simulink library "speedgoatlib_IO622"  (R2024b)
settings: Solver=ode45  StartTime=0.0  StopTime=10.0  RelTol=1e-3  EnableMultiTasking=on
libraries: slrealtimeethercatlib x10, simulink x4, simulink_extras x2
Description:
  | 7.14.0.739 (R2012a)
settings Model: sg_rtwmakecfg_data=_sglibc_  Creator=dkuratli  LastModifiedBy=speedgoat\jenkins
settings SolverCC: AlgebraicLoopSolver=TrustRegion
settings DataIOCC: LimitDataPoints=on  SaveFormat=Array  SignalLoggingSaveFormat=ModelDataLogs  ReturnWorkspaceOutputs=off
settings OptimizationCC: ReuseModelBlockBuffer=off  ExpressionDepthLimit=2147483647  LifeSpan=inf
settings DebuggingCC: UnderspecifiedInitializationDetection=Classic  MergeDetectMultiDrivingBlocksExec=none  SolverPrmCheckMsg=warning  FcnCallInpInsideContextMsg=warning  UnconnectedInputMsg=warning  UnconnectedOutputMsg=warning  UnconnectedLineMsg=warning  AllowSymbolicDim=off  StateNameClashWarn=warning  PregeneratedLibrarySubsystemCodeDiagnostic=none  SFUnexpectedBacktrackingDiag=warning  SFNoUnconditionalDefaultTransitionDiag=warning  SFExecutionAtInitializationDiag=none  ArithmeticOperatorsInVariantConditions=warning
settings HardwareCC: ProdBitPerPointer=32  ProdBitPerSizeT=32  ProdBitPerPtrDiffT=32  ProdLargestAtomicFloat=None  ProdIntDivRoundTo=Undefined  ProdEndianess=Unspecified  ProdWordSize=32  ProdHWDeviceType=32-bit Generic
settings ModelReferenceCC: EnableRefExpFcnMdlSchedulingChecks=on  PropagateSignalLabelsOutOfModel=off
settings SFSimCC: SimUseLocalCustomCode=off  CustomCodeUndefinedFunction=UseInterfaceOnly
settings RTWCC: RTWUseLocalCustomCode=off  GPUComputeCapability=3.5  DLArmComputeVersion=19.05
settings CodeAppCC: StateflowObjectComments=on
settings GRTTargetCC: TargetLangStandard=C89/C90 (ANSI)  CombineOutputUpdateFcns=off  GRTInterface=on
settings ConfigComp: CovMetricSettings=dw  CovSaveCumulativeToWorkspaceVar=on  CovSaveSingleToWorkspaceVar=on  CovExternalEMLEnable=off  CovSFcnEnable=off  CovBoundaryAbsTol=1.0e-5

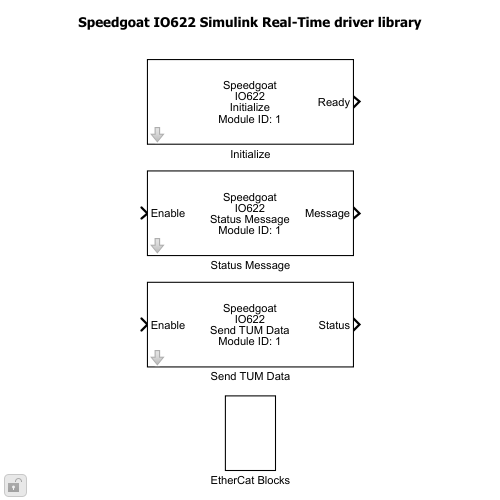
[thumbnail: Simulink's stored preview of the top-level diagram]
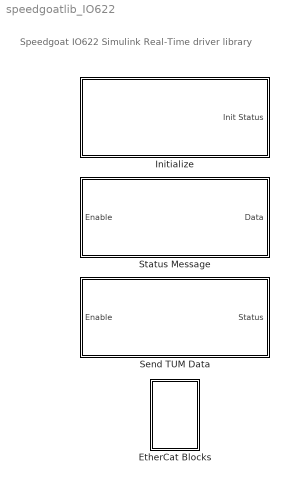
== system speedgoatlib_IO622 ==
  note: Speedgoat IO622 Simulink Real-Time driver library
  EtherCat Blocks : Subsystem
      settings: OpenFcn=|
      | if sg.utils.isSlrealtimeRelease
      | slrealtimeethercatlib
      | else
      | xpcethercatlib
      | end
  Initialize : Subsystem  InitFcn=|  mask(init_IO622){parModuleId=1, parSlaveName=<empty>, parSlaveAddr=[], parFirmwarePath=, parTs=-1}
      | sg.block.init();
      | 
      | sg_IO622_init(1);
      mask prompts: parModuleId "IO622 Module Identifier"; parSlaveName "EB Box"; parSlaveAddr "EB Box Address"; parFirmwarePath "Firmware Path"; parTs "Sample Time"
      mask help: Speedgoat driver block<br>IO622 - Initialize<br><br>&copy; 2007 - 2017, Speedgoat GmbH, www.speedgoat.com
      mask init:
      | sg_IO622_init(3);
      mask Help: eval('sg.utils.help.show({''io_main/refentry_ref_IO622''});')
      mask TypeOptions parModuleId: 1 | 2 | 3 | 4 | 5 | 6 | 7 | 8 | 9 | 10
      mask Callback parModuleId: sg_IO622_init(2,1)
      mask TypeOptions parSlaveName: <empty>
      mask Callback parSlaveName: sg_IO622_init(2,2)
      mask DialogControl Container3 Prompt: Module Settings
      mask DialogControl Container4 Prompt: EB Box Settings
      mask Display: disp('Speedgoat\nIO622\nInitialize\nModule ID: 1');port_label('output',1,'Ready');
  Send TUM Data : Subsystem  InitFcn=|  mask(send_IO622){parModuleId=1, parConfigFile=, parSlaveName=<empty>, parSlaveAddr=[], parSampleTime=-1, parTUMfunction=<empty>, parTUMid=0, parTUMinstance=<empty>, parTUMmode=<empty>, parModeId=0, parTUMoffset=0, parTUMlength=0, parTUMdataType=0, parByteGroupId=0, parSignal=<empty>, parSignalId=0, parSignalData=<empty>, parNumInputs=0, parNameInputs=<empty>, parTUMdata=0}
      | sg.block.init();
      | 
      | sg_IO622_tum(1);
      mask prompts: parModuleId "IO622 Module Identifier"; parConfigFile "Database File"; parSlaveName "EB Box"; parSlaveAddr "EB Box Address"; parSampleTime "Sample Time"; parTUMfunction "TUM Function"; parTUMid "TUM function id"; parTUMinstance "TUM Instance"; parTUMmode "TUM Mode"; parModeId "TUM mode id"; parTUMoffset "TUM data offset"; parTUMlength "TUM data length"; parTUMdataType "TUM data type"; parByteGroupId "TUM byte group id"; parSignal "Signal"; parSignalId "Signal id"; parSignalData "Termination"; parNumInputs "Number of Inputs"; parNameInputs "Name of Inputs"; parTUMdata "TUM data"
      mask help: Speedgoat driver block<br>IO622 - Send TUM Data<br><br>&copy; 2007 - 2017, Speedgoat GmbH, www.speedgoat.com
      mask init:
      | sg_IO622_tum(3);
      mask Help: eval('sg.utils.help.show({''io_main/refentry_ref_IO622''});')
      mask TypeOptions parModuleId: 1 | 2 | 3 | 4 | 5 | 6 | 7 | 8 | 9 | 10
      mask Callback parModuleId: sg_IO622_tum(2,1)
      mask Callback parConfigFile: sg_IO622_tum(2,2)
      mask TypeOptions parTUMfunction: <empty>
      mask Callback parTUMfunction: sg_IO622_tum(2,4)
      mask TypeOptions parTUMinstance: <empty>
      mask TypeOptions parTUMmode: <empty>
      mask Callback parTUMmode: sg_IO622_tum(2,5)
      mask TypeOptions parSignal: <empty>
      mask Callback parSignal: sg_IO622_tum(2,6)
      mask TypeOptions parSignalData: <empty>
      mask Callback parSignalData: sg_IO622_tum(2,7)
      mask TypeOptions parNameInputs: <empty>
      mask DialogControl Container4 Prompt: Module Settings
      mask DialogControl Control2 Prompt: Browse
      mask DialogControl Control2 Callback: sg_IO622_tum(2,3)
      mask DialogControl Container3 Prompt: TUM Settings
      mask Display: disp('Speedgoat\nIO622\nSend TUM Data\nModule ID: 1');port_label('output',1,'Status');port_label('input',1,'Enable');
  Status Message : Subsystem  InitFcn=|  mask(status_IO622){parModuleId=1, parSlaveName=<empty>, parSlaveAddr=[], parDispInfo=on, parDispWarning=on, parDispError=on, parDebugMsg=off}
      | sg.block.init();
      | 
      | sg_IO622_status(1);
      mask prompts: parModuleId "IO622 Module Identifier"; parSlaveName "EB Box"; parSlaveAddr "EB Box Address"; parDispInfo "Display Info"; parDispWarning "Display Warnings"; parDispError "Display Error"; parDebugMsg "Enable Message Output (Increased Execution Time)"
      mask help: Speedgoat Driver Block<br>IO622 - Status Message<br><br>&copy; 2007 - 2023, Speedgoat GmbH, <a href="matlab: web('www.speedgoat.com','-browser');">www.speedgoat.com</a>
      mask init:
      | sg_IO622_status(3);
      mask Help: eval('sg.utils.help.show(''io_main/refentry_ref_io622'');')
      mask TypeOptions parModuleId: 1 | 2 | 3 | 4 | 5 | 6 | 7 | 8 | 9 | 10
      mask Callback parModuleId: sg_IO622_status(2);
      mask DialogControl Container4 Prompt: Module Settings
      mask DialogControl Container5 Prompt: Status Message Settings
      mask DialogControl Container6 Prompt: Target Console
      mask Display: disp('Speedgoat\nIO622\nStatus Message\nModule ID: 1');port_label('input',1,'Enable');port_label('output',1,'Message');

== system speedgoatlib_IO622/EtherCat Blocks ==

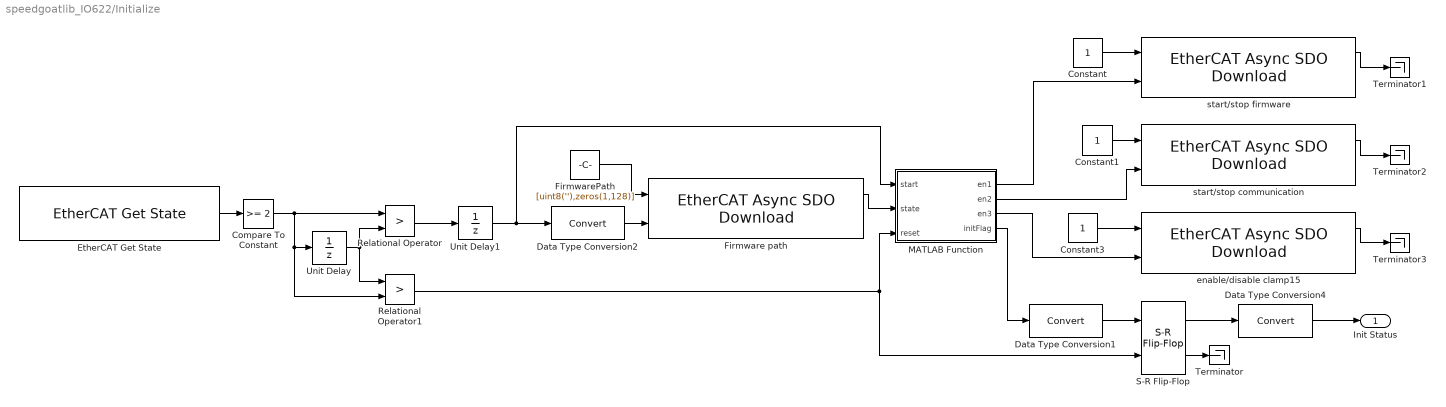
== system speedgoatlib_IO622/Initialize ==
  Compare To Constant : simulink/Logic and Bit Operations/Compare To Constant  relop=>=  const=2  OutDataTypeStr=boolean
  Constant : Constant  OutDataTypeStr=Inherit: Inherit via back propagation
  Constant1 : Constant  OutDataTypeStr=Inherit: Inherit via back propagation
  Constant3 : Constant  OutDataTypeStr=Inherit: Inherit via back propagation
  Data Type Conversion1 : DataTypeConversion  SaturateOnIntegerOverflow=off  RndMeth=Floor
  Data Type Conversion2 : DataTypeConversion  SaturateOnIntegerOverflow=off  RndMeth=Floor
  Data Type Conversion4 : DataTypeConversion  SaturateOnIntegerOverflow=off  RndMeth=Floor
  "EtherCAT Get State  " : slrealtimeethercatlib/EtherCAT Get State  device_id=1  sample_time=-1
  Firmware path : slrealtimeethercatlib/EtherCAT Async SDO Download  index=20512  subIndex=1  sig_type=uint8  sig_dim=128  device_id=1  subdevice_name=<empty>  sample_time=-1  subdevice_addr=[]  selected_subdevice=Term 1 (EK1100)  timeout=500  subdevice_found=0  complete=0
  FirmwarePath : Constant  Value=[uint8(''),zeros(1,128)]  OutDataTypeStr=Inherit: Inherit via back propagation
  MATLAB Function : MATLAB Function  TreatAsAtomicUnit=on
  Relational Operator : RelationalOperator  Operator=>  OutDataTypeStr=boolean  RndMeth=Simplest  InputSameDT=off
  Relational Operator1 : RelationalOperator  Operator=>  OutDataTypeStr=boolean  RndMeth=Simplest  InputSameDT=off
  S-R Flip-Flop : simulink_extras/Flip Flops/S-R Flip-Flop  initial_condition=0
  Terminator{,1..3} (4 alike) : Terminator
  Unit Delay : UnitDelay  SampleTime=-1
  Unit Delay1 : UnitDelay  SampleTime=-1
  enable/disable clamp15 : slrealtimeethercatlib/EtherCAT Async SDO Download  index=20512  subIndex=4  sig_type=boolean  sig_dim=1  device_id=1  subdevice_name=<empty>  sample_time=-1  subdevice_addr=[]  selected_subdevice=Term 1 (EK1100)  timeout=500  subdevice_found=0  complete=0
  start/stop communication : slrealtimeethercatlib/EtherCAT Async SDO Download  index=20512  subIndex=3  sig_type=boolean  sig_dim=1  device_id=1  subdevice_name=<empty>  sample_time=-1  subdevice_addr=[]  selected_subdevice=Term 1 (EK1100)  timeout=500  subdevice_found=0  complete=0
  start/stop firmware : slrealtimeethercatlib/EtherCAT Async SDO Download  index=20512  subIndex=2  sig_type=boolean  sig_dim=1  device_id=1  subdevice_name=<empty>  sample_time=-1  subdevice_addr=[]  selected_subdevice=Term 1 (EK1100)  timeout=500  subdevice_found=0  complete=0
  Init Status : Outport  VectorParamsAs1DForOutWhenUnconnected=off
  wires:
  FirmwarePath/1 -> Firmware path/1
  Constant/1 -> start/stop firmware/1
  Constant1/1 -> start/stop communication/1
  Firmware path/1 -> MATLAB Function/2(state)
  Constant3/1 -> enable/disable clamp15/1
  "EtherCAT Get State  "/1 -> Compare To Constant/1
  Unit Delay/1 -> Relational Operator1/1, Relational Operator/2
  Compare To Constant/1 -> Relational Operator/1, Relational Operator1/2, Unit Delay/1
  Relational Operator/1 -> Unit Delay1/1
  Unit Delay1/1 -> Data Type Conversion2/1, MATLAB Function/1(start)
  S-R Flip-Flop/2 -> Terminator/1
  S-R Flip-Flop/1 -> Data Type Conversion4/1
  MATLAB Function/4(initFlag) -> Data Type Conversion1/1
  Relational Operator1/1 -> S-R Flip-Flop/2, MATLAB Function/3(reset)
  Data Type Conversion1/1 -> S-R Flip-Flop/1
  start/stop firmware/1 -> Terminator1/1
  enable/disable clamp15/1 -> Terminator3/1
  start/stop communication/1 -> Terminator2/1
  Data Type Conversion4/1 -> Init Status/1
  Data Type Conversion2/1 -> Firmware path/2
  MATLAB Function/3(en3) -> enable/disable clamp15/2
  MATLAB Function/1(en1) -> start/stop firmware/2
  MATLAB Function/2(en2) -> start/stop communication/2

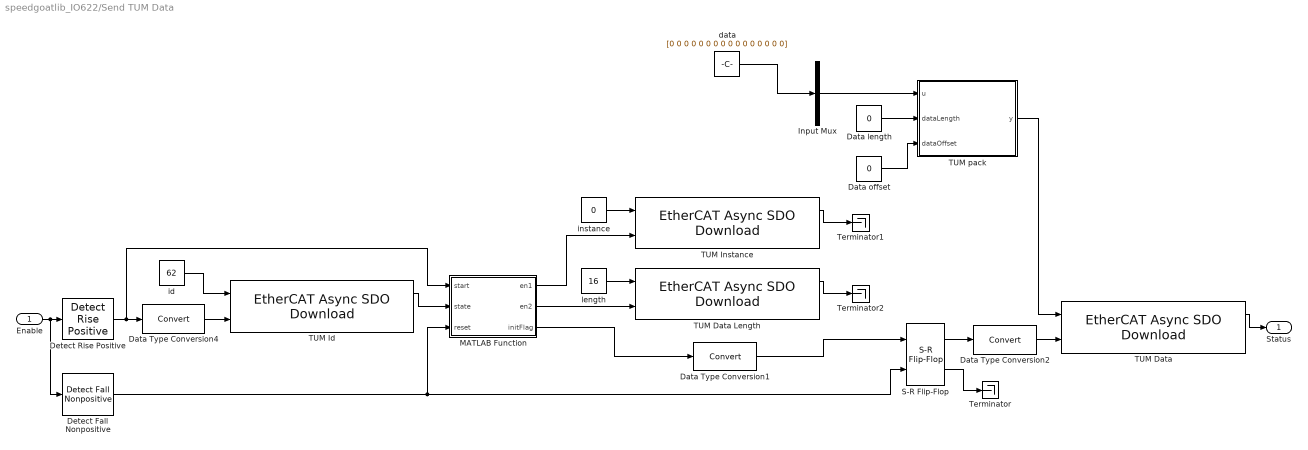
== system speedgoatlib_IO622/Send TUM Data ==
  Enable : Inport
  Data Type Conversion1 : DataTypeConversion  SaturateOnIntegerOverflow=off  RndMeth=Floor
  Data Type Conversion2 : DataTypeConversion  SaturateOnIntegerOverflow=off  RndMeth=Floor
  Data Type Conversion4 : DataTypeConversion  SaturateOnIntegerOverflow=off  RndMeth=Floor
  Data length : Constant  Value=0
  Data offset : Constant  Value=0
  Detect Fall Nonpositive : simulink/Logic and Bit Operations/Detect Fall Nonpositive  vinit=1  OutDataTypeStr=boolean
  Detect Rise Positive : simulink/Logic and Bit Operations/Detect Rise Positive  vinit=0  OutDataTypeStr=boolean
  Input Mux : Mux  Inputs=1
  MATLAB Function : MATLAB Function  TreatAsAtomicUnit=on
  S-R Flip-Flop : simulink_extras/Flip Flops/S-R Flip-Flop  initial_condition=0
  TUM Data : slrealtimeethercatlib/EtherCAT Async SDO Download  index=20480  subIndex=4  sig_type=uint8  sig_dim=16  device_id=1  subdevice_name=<empty>  sample_time=-1  subdevice_addr=[]  selected_subdevice=Term 1 (EK1100)  timeout=500  subdevice_found=1  complete=0
  TUM Data Length : slrealtimeethercatlib/EtherCAT Async SDO Download  index=20480  subIndex=3  sig_type=uint16  sig_dim=1  device_id=1  subdevice_name=<empty>  sample_time=-1  subdevice_addr=[]  selected_subdevice=Term 1 (EK1100)  timeout=500  subdevice_found=1  complete=0
  TUM Id : slrealtimeethercatlib/EtherCAT Async SDO Download  index=20480  subIndex=1  sig_type=uint16  sig_dim=1  device_id=1  subdevice_name=<empty>  sample_time=-1  subdevice_addr=[]  selected_subdevice=Term 1 (EK1100)  timeout=500  subdevice_found=1  complete=0
  TUM Instance : slrealtimeethercatlib/EtherCAT Async SDO Download  index=20480  subIndex=2  sig_type=uint16  sig_dim=1  device_id=1  subdevice_name=<empty>  sample_time=-1  subdevice_addr=[]  selected_subdevice=Term 1 (EK1100)  timeout=500  subdevice_found=1  complete=0
  TUM pack : MATLAB Function  TreatAsAtomicUnit=on
  Terminator : Terminator
  Terminator1 : Terminator
  Terminator2 : Terminator
  data : Constant  Value=[0 0 0 0 0 0 0 0 0 0 0 0 0 0 0 0]  OutDataTypeStr=double
  id : Constant  Value=62  OutDataTypeStr=Inherit: Inherit via back propagation
  instance : Constant  Value=0  OutDataTypeStr=Inherit: Inherit via back propagation
  length : Constant  Value=16  OutDataTypeStr=Inherit: Inherit via back propagation
  Status : Outport  VectorParamsAs1DForOutWhenUnconnected=off
  wires:
  id/1 -> TUM Id/1
  instance/1 -> TUM Instance/1
  length/1 -> TUM Data Length/1
  Data Type Conversion2/1 -> TUM Data/2
  TUM Data/1 -> Status/1
  Data Type Conversion4/1 -> TUM Id/2
  Enable/1 -> Detect Fall Nonpositive/1, Detect Rise Positive/1
  Detect Rise Positive/1 -> MATLAB Function/1(start), Data Type Conversion4/1
  S-R Flip-Flop/1 -> Data Type Conversion2/1
  Detect Fall Nonpositive/1 -> MATLAB Function/3(reset), S-R Flip-Flop/2
  Input Mux/1 -> TUM pack/1(u)
  data/1 -> Input Mux/1
  Data offset/1 -> TUM pack/3(dataOffset)
  Data length/1 -> TUM pack/2(dataLength)
  S-R Flip-Flop/2 -> Terminator/1
  TUM Id/1 -> MATLAB Function/2(state)
  MATLAB Function/1(en1) -> TUM Instance/2
  MATLAB Function/3(initFlag) -> Data Type Conversion1/1
  MATLAB Function/2(en2) -> TUM Data Length/2
  TUM Instance/1 -> Terminator1/1
  TUM Data Length/1 -> Terminator2/1
  Data Type Conversion1/1 -> S-R Flip-Flop/1
  TUM pack/1(y) -> TUM Data/1

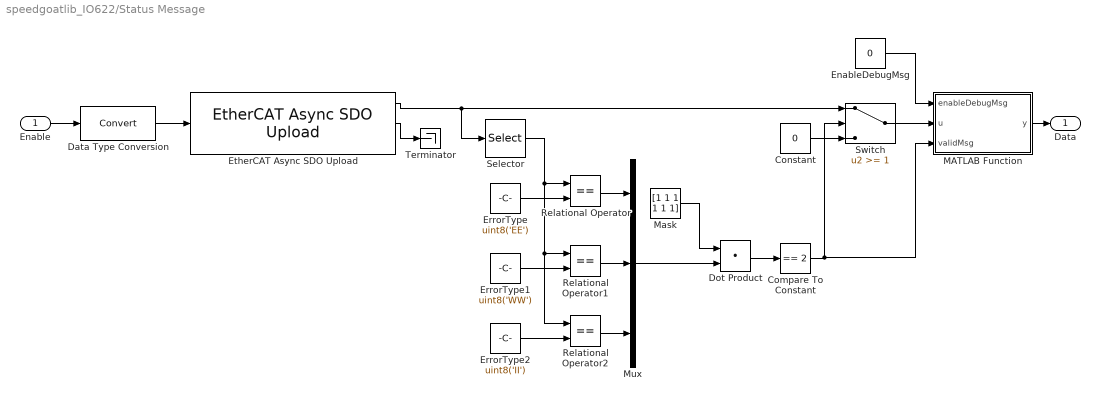
== system speedgoatlib_IO622/Status Message ==
  Enable : Inport
  Compare To Constant : simulink/Logic and Bit Operations/Compare To Constant  relop===  const=2  OutDataTypeStr=boolean
  Constant : Constant  Value=0  OutDataTypeStr=uint8
  Data Type Conversion : DataTypeConversion  SaturateOnIntegerOverflow=off  RndMeth=Floor
  Dot Product : DotProduct  OutDataTypeStr=Inherit: Inherit via internal rule
  EnableDebugMsg : Constant  Value=0  OutDataTypeStr=uint8
  ErrorType : Constant  Value=uint8('EE')
  ErrorType1 : Constant  Value=uint8('WW')
  ErrorType2 : Constant  Value=uint8('II')
  EtherCAT Async SDO Upload : slrealtimeethercatlib/EtherCAT Async SDO Upload  index=20560  subIndex=1  sig_type=uint8  sig_dim=256  device_id=1  subdevice_name=<empty>  sample_time=-10  subdevice_addr=[]  selected_subdevice=Term 1 (EK1100)  timeout=500  subdevice_found=1  complete=0
  MATLAB Function : MATLAB Function  TreatAsAtomicUnit=on
  Mask : Constant  Value=[1 1 1 1 1 1]  OutDataTypeStr=Inherit: Inherit via back propagation
  Mux : Mux  Inputs=3
  Relational Operator : RelationalOperator  Operator===  OutDataTypeStr=boolean  RndMeth=Simplest  InputSameDT=off
  Relational Operator1 : RelationalOperator  Operator===  OutDataTypeStr=boolean  RndMeth=Simplest  InputSameDT=off
  Relational Operator2 : RelationalOperator  Operator===  OutDataTypeStr=boolean  RndMeth=Simplest  InputSameDT=off
  Selector : Selector  InputPortWidth=256  IndexOptions=Index vector (dialog)  Indices=[2:3]  OutputSizes=1
  Switch : Switch  Threshold=1  SaturateOnIntegerOverflow=off  InputSameDT=off
  Terminator : Terminator
  Data : Outport  VectorParamsAs1DForOutWhenUnconnected=off
  wires:
  Enable/1 -> Data Type Conversion/1
  EtherCAT Async SDO Upload/1 -> Switch/1, Selector/1
  ErrorType/1 -> Relational Operator/2
  Selector/1 -> Relational Operator/1, Relational Operator1/1, Relational Operator2/1
  Constant/1 -> Switch/3
  ErrorType1/1 -> Relational Operator1/2
  ErrorType2/1 -> Relational Operator2/2
  EtherCAT Async SDO Upload/2 -> Terminator/1
  Relational Operator/1 -> Mux/1
  Relational Operator1/1 -> Mux/2
  Relational Operator2/1 -> Mux/3
  Mask/1 -> Dot Product/1
  Mux/1 -> Dot Product/2
  Compare To Constant/1 -> MATLAB Function/3(validMsg), Switch/2
  Dot Product/1 -> Compare To Constant/1
  Data Type Conversion/1 -> EtherCAT Async SDO Upload/1
  Switch/1 -> MATLAB Function/2(u)
  MATLAB Function/1(y) -> Data/1
  EnableDebugMsg/1 -> MATLAB Function/1(enableDebugMsg)

== matlab function speedgoatlib_IO622/Initialize/MATLAB Function ==
  data: start input; state input; en1 output; en2 output; en3 output; initFlag output; reset input
function [en1,en2,en3,initFlag] = fcn(start,state,reset)

    persistent sendCnt oldState enable;
    
    if isempty(oldState)
        oldState=int32(0);
    end
    if isempty(sendCnt)
        sendCnt=1;
    end
    if isempty(enable)
        enable=0;
    end
    
    if reset == 1
        sendCnt=1;
        enable=0;
    end
    
    en1=int32(0); en2=int32(0); en3=int32(0); initFlag=int32(0);
    if start == 1
        enable=1;
    end
    
    if enable == 1
        if sendCnt<=4
            if oldState == 2 && state == 0
                switch(sendCnt)
                    case 1
                        en1=int32(1);
                    case 2
                        en2=int32(1);
                    case 3
                        en3=int32(1);  
                    case 4
                        initFlag=int32(1);
                    otherwise
                        %error('SendCnt overflow');
                end
                sendCnt=sendCnt+1;
            end
        end
    end
    
    oldState = state;
end

== matlab function speedgoatlib_IO622/Send TUM Data/TUM pack ==
  data: u input; y output uint8; dataLength input; dataOffset input
function y = pack(u,dataLength,dataOffset)

    tempData=zeros(1,8,'uint8');
    y=zeros(16,1,'uint8');
    
    %insert basic data
    y=uint8(u(1:16));
    %pack data if required
    if length(u) > 16
        for i=17:length(u)
            tempData=typecast(int64(u(i)),'uint8');
            for j=0:dataLength(i-16)-1
                y(j+dataOffset(i-16))=tempData(dataLength(i-16)-j);
            end
        end
    end

end

== matlab function speedgoatlib_IO622/Send TUM Data/MATLAB Function ==
  data: start input; state input; en1 output; en2 output; initFlag output; reset input
function [en1,en2,initFlag] = fcn(start,state,reset)

    persistent sendCnt oldState enable;
    
    if isempty(oldState)
        oldState=int32(0);
    end
    if isempty(sendCnt)
        sendCnt=1;
    end
    if isempty(enable)
        enable=0;
    end
    
    en1=int32(0); en2=int32(0); initFlag=int32(0);
    if start == 1
        enable=1;
    end
    
    if reset == 1
        sendCnt=1;
        enable=0;
    end
    
    if enable == 1
        if sendCnt<=3
            if oldState == 2 && state == 0
                switch(sendCnt)
                    case 1
                        en1=int32(1);
                    case 2
                        en2=int32(1);
                    case 3
                        initFlag=int32(1);
                    otherwise
                        %error('SendCnt overflow');
                end
                sendCnt=sendCnt+1;
            end
        end
    end
    
    oldState = state;
end

== matlab function speedgoatlib_IO622/Status Message/MATLAB Function ==
  data: enableDebugMsg input; u input; y output; validMsg input
function y = fcn(enableDebugMsg, u, validMsg)

    if (enableDebugMsg&&validMsg)
        fprintf('%s\n',deblank(char(u)));
    end
    
y = u;
